simulink library "m3_common_lib"  (R2021b)
settings: Solver=ode45  StartTime=0.0  StopTime=10.0  RelTol=1e-3
undefined symbols (not defined in the file or in its folder): ACCEL_PRE_MULT, APDT_SrvcMgr_IRVHVDCSubFcnReq, C_C1GearNumbers, C_C1GearRatios, C_Calibration, C_DitherWaveform, C_GearOffset, C_GearRatioIn, C_GearRatioInverseOut, C_GearRatioOut, CLUTCH_INNER_LOOP_UPDATE_RATE, CONSTANT, DEGRADED_MODE_SIZE, Dem_EventStatusType, DiscIntNeverNeededParam, F_FAULT_ENUM, F_NOFAULT, F_OUTOFRANGE, F_RATELIMIT, FALSE, FMI14_SPECIAL_INSTRUCTIONS, FMI20_DATA_DRIFTED_HIGH, FMI21_DATA_DRIFTED_LOW, FMI29_RESERVED_FOR_SAE_ASSIGNMENT, FMI30_RESERVED_FOR_SAE_ASSIGNMENT, FMI31_CONDITION_EXISTS, FMI32_NO_FAULT, IC, k_accel, k_mean, MAX_UINT32, MEAN_PRE_MULT, NTriggers, QLTY_SIGNAL_FAILED, QLTY_SIGNAL_FULLY_FUNCTION, QLTY_SIGNAL_SUBSTITUTED_BY_1ST_CHOICE, QLTY_SIGNAL_SUBSTITUTED_BY_2ND_CHOICE, QLTY_SIGNAL_SUBSTITUTED_BY_3RD_CHOICE, QLTY_SIGNAL_SUBSTITUTED_BY_4TH_CHOICE, SAMPLE_TIME_100us, simin, T_TestPoint, TF_FALSE, TF_TRUE, TimeStep, TRUE, WORKSPACE_UPDATE_RATE, Zero, ZERO
libraries: $bdroot x121, simulink x23, simulink_extras x4, MBD_EPS_Local_Blockset x4
(part 2 of 10)

== system m3_common_lib/Diagnostics ==
  note: DEPRECATED
  note: Diagnostics
  note: DEPRECATED
  Calibration Enabled Debounce : Subsystem
      settings: RTWSystemCode=Inline
  Calibration Enabled Debounce Boolean Input : Subsystem
      settings: RTWSystemCode=Inline
  Calibration Enabled MinMax OOR : Subsystem  mask(Calibration Enabled OOR Detection Subsystem){InitialValue=0, InDataType=single}
      mask prompts: InitialValue "Initial Value"; InDataType "Input Data Type"
      mask init:
      | DataType = get_param(gcb, 'InDataType');
      | OOR = [gcb '/Enabled OOR'];
      | 
      | set_param(OOR, 'InDataType', DataType);
      mask TypeOptions InDataType: single | int16
  Calibration Enabled MinMax RLim : Subsystem  mask(Calibration Enabled RateLimit Detection Subsystem){IC=0, TimeStep=TimeStep, InDataType=single}
      mask prompts: IC "Initial Condition"; TimeStep "Update Time"; InDataType "Input Data Type"
      mask init:
      | DataType = get_param(gcb, 'InDataType');
      | RLim = [gcb '/Enabled RLim'];
      | 
      | set_param(RLim, 'InDataType', DataType);
      mask TypeOptions InDataType: single | int16
  Ccaller_DiagLv1 : Subsystem  TreatAsAtomicUnit=on
      settings: RTWSystemCode=Nonreusable function
  Ccaller_DiagLv2 : Subsystem  TreatAsAtomicUnit=on
      settings: RTWSystemCode=Nonreusable function
  DiagFaultCounter : Subsystem
  ExtractValue : Subsystem
      mask Display:
      | patch([0.3 0.3 0.7 0.7], [0.4 0.6 0.6 0.4], [205/255 205/255 255/255]);
      | disp('FromInputSignal')
      | port_label('input', 1, 'in');
      | port_label('output', 1, 'value');
      | port_label('output', 2, 'FMI');
  FMIUpdate : Subsystem
  Fault Debounce Lv1 Boolean Input : Subsystem
  Fault Debounce Lv1 state Input : Subsystem
  FaultStatusUpdate : Subsystem
  KeepAlive : Subsystem  TreatAsAtomicUnit=on  mask(KeepAlive){Operator===, UseSigObject=off}
      mask prompts: Operator "Relational Operator"; UseSigObject "Reuse Signal Object for Unit Delay"
      mask help:
      | Use to enable a subsystem that needs to keep itself alive based on a state created by the block.
      |
      | Enable = KeepAlive || (A (RelOp) B)
      |
      | Where RelOp can be any of the relational operators.
      | A and B must have the same data type.
      | All inputs must be scalars.
      |
      | Second output is the value of the (A (RelOp) B) which could be used in the enabled subsystem or for logging or terminated if unneeded.
      |
      | Checking "Reuse Signal Object for Unit Delay" is an optimization for when the signal driving KeepAlive is already a signal object.  Instead of allocating new memory for the unit delay, the unit delay will use the signal object.  In this case do not set the driving signal to "Resolve to Signal Object".
      mask init:
      | set_param([gcb '/RelOp'],'Operator',get_param(gcb,'Operator'));
      | 
      | ud = get_param([gcb '/Delay'],'Object');
      | if UseSigObject
      | st = get_param([gcb '/State'],'Object');
      | lh = st.PortHandles.Outport;
      | set(lh,'ShowPropagatedSignals','on');
      | set(lh,'ShowPropagatedSignals','off');
      | set(lh,'ShowPropagatedSignals','on');
      | sigName = get(lh,'PropagatedSignals');
      | ud.StateName = sigName;
      | ud.StateMustResolveToSignalObject = 'on';
      | else
      | ud.StateName = '';
      | ud.StateMustResolveToSignalObject = 'off';
      | end
      settings: RTWSystemCode=Inline
      mask TypeOptions Operator: == | ~= | < | <= | >= | >
      mask Display:
      | patch([0.3 0.3 0.7 0.7], [0.35 0.65 0.65 0.35], [255/255 127/255 255/255]);
      | 
      | if ~UseSigObject
      |    port_label('input',1,'KeepAlive');
      | else
      |    ph = get_param([gcb '/State'],'PortHandles');
      |    sigName = get(ph.Outport,'PropagatedSignals');
      |    port_label('input',1,['-E ' sigName]);
      | end
      | port_label('input',2,'A');
      | port_label('input',3,'B');
      | port_label('output',1,'Enable');
      | port_label('output',2,sprintf('(A %s B)',get_param(gcb,'Operator')));
  LogicBasedActivation : Subsystem  mask(AddDegradedMode){DM_SIZE=DEGRADED_MODE_SIZE}
      mask prompts: DM_SIZE "Degraded Mode Vector Size"
      mask help:
      | Logic based activation adds additional degraded modes if Add? input is true.  The logic can be disabled by the Enable input.
      |
      | - Enable: Allow or disallow logic.  Should be constant or calibration.
      | - DMToAdd: Packed degraded modes to add.  Size must match "Degraded Mode Vector Size" parameter.
      | - Add?: Boolean input to add DMs or pass through DMPackedData unchanged.
      | - DMPackedData: Current set of degraded modes.
      mask Display:
      | patch([0.3 0.3 0.7 0.7], [0.35 0.65 0.65 0.35], [255/255 127/255 255/255]);
      | port_label('input',1,'Enable');
      | port_label('input',2,'DMToAdd');
      | port_label('input',3,'Add?');
      | port_label('input',4,'DMPackedData');
      | port_label('output',1,'DMPackedData');
  LogicBasedDeactivation : Subsystem  mask(RemoveDegradedMode){DM_SIZE=DEGRADED_MODE_SIZE}
      mask prompts: DM_SIZE "Degraded Mode Vector Size"
      mask help:
      | Logic based deactivation removes degraded modes if Remove? input is true.  The logic can be disabled by the Enable input.
      |
      | - Enable: Allow or disallow logic.  Should be constant or calibration.
      | - DMToRemove: Packed degraded modes to remove.  Size must match "Degraded Mode Vector Size" parameter.
      | - Remove?: Boolean input to remove DMs or pass through DMPackedData unchanged.
      | - DMPackedData: Current set of degraded modes.
      mask Display:
      | patch([0.3 0.3 0.7 0.7], [0.35 0.65 0.65 0.35], [255/255 127/255 255/255]);
      | port_label('input',1,'Enable');
      | port_label('input',2,'DMToRemove');
      | port_label('input',3,'Remove?');
      | port_label('input',4,'DMPackedData');
      | port_label('output',1,'DMPackedData');
  OOR Fault Detect Enum : Subsystem  RTWFcnName=OOR  mask(CL OOR Fault Detection with Enable){InitialValue=0, k_min=0, k_max=0}
      mask prompts: InitialValue "Initial Value"; k_min "Lower Limit"; k_max "Upper Limit"
      mask help:
      | Out of range fault detection block with enable for Enum signals
      |
      | X(1) = input signal
      | X(2) = enable
      |
      | Y(1) = output signal
      | Y(2) = fault indication
      settings: RTWSystemCode=Inline  RTWFcnNameOpts=User specified  RTWFileNameOpts=Use function name
      mask Help: web(which(['common_lib12.html']))
      mask Display:
      | patch([0.1 0.1 0.9 0.9], [0.35 0.65 0.65 0.35], [255/255 127/255 255/255])
      | %disp('OOR/En')
      | 
      | min=get_param(gcb,'k_min')
      | max=get_param(gcb,'k_max')
      | 
      | txt = sprintf('\tUpper Lim: %s\n\tLower Lim: %s',max,min);
      | disp(txt)
      | 
      | port_label('input',1,'in')
      | port_label('input',2,'enable')
      | port_label('output',1,'out')
      | port_label('output',2,'fault?')
  OOR Fault Detection : Subsystem  RTWFcnName=OOR  mask(CL OOR Fault Detection with Enable){InitialValue=0, k_min=0, k_max=0, applyLimits=0}
      mask prompts: InitialValue "Initial Value"; k_min "Upper Limit"; k_max "Lower Limit"
      mask help:
      | Out of range fault detection block with enable
      |
      | X(1) = input signal
      | X(2) = enable
      |
      | Y(1) = saturated out
      | Y(2) = fault indication
      mask init:
      | portNumber = 1;
      | outMin = [];
      | outMax = [];
      | portHandles = get_param(gcb,'PortHandles');
      | inportHandle = portHandles.Inport(portNumber);
      | lineHandle = get_param(inportHandle,'Line');
      | if(lineHandle>0) 
      |     nvSrcPorts = get_param(lineHandle, 'NonVirtualSrcPorts');
      |     nvLineHandle = get_param(nvSrcPorts, 'line');
      |     if(nvLineHandle>0)
      |         nvSrcBlkHandle = get_param(nvLineHandle, 'SrcBlockHandle'); 
      |         blockTypeStr = get_param(nvSrcBlkHandle, 'BlockType');
      |         if(strcmp(blockTypeStr,'Inport')>0)
      |             outMin = get_param(nvSrcBlkHandle, 'OutMin');
      |             outMax = get_param(nvSrcBlkHandle, 'OutMax');
      |             set_param(gcb,'k_min',outMin);
      |             set_param(gcb,'k_max',outMax);
      |         else
      |             set_param(gcb,'k_min','0');
      |             set_param(gcb,'k_max','0');
      |             outMin = [];
      |             outMax = [];
      |         end
      |     else
      |         set_param(gcb,'k_min','0');
      |         set_param(gcb,'k_max','0');
      |         outMin = [];
      |         outMax = [];
      |     end
      | else
      |     set_param(gcb,'k_min','0');
      |     set_param(gcb,'k_max','0');
      |     outMin = [];
      |     outMax = [];
      | end
      | 
      | 
      | if isempty(outMin) || isempty(outMax) || ((strcmp(outMin,'0')>0)&&(strcmp(outMin,'0')>0))
      |     %applyLimits=false;
      |     set_param(gcb,'applyLimits','0')
      | else
      |     set_param(gcb,'applyLimits','1')
      | end
      settings: RTWSystemCode=Inline  RTWFcnNameOpts=User specified  RTWFileNameOpts=Use function name
      mask Help: web(which(['common_lib12.html']))
      mask DialogControl Control2 Prompt: Update
      mask DialogControl Control2 Callback:
      | portNumber = 1;
      | outMin = [];
      | outMax = [];
      | portHandles = get_param(gcb,'PortHandles');
      | inportHandle = portHandles.Inport(portNumber);
      | lineHandle = get_param(inportHandle,'Line');
      | if(lineHandle>0)
      |     nvSrcPorts = get_param(lineHandle, 'NonVirtualSrcPorts');
      |     nvLineHandle = get_param(nvSrcPorts, 'line');
      |     if(nvLineHandle>0)
      |         nvSrcBlkHandle = get_param(nvLineHandle, 'SrcBlockHandle');
      |         blockTypeStr = get_param(nvSrcBlkHandle, 'BlockType');
      |         if(strcmp(blockTypeStr,'Inport')>0)
      |             outMin = get_param(nvSrcBlkHandle, 'OutMin');
      |             outMax = get_param(nvSrcBlkHandle, 'OutMax');
      |             set_param(gcb,'k_min',outMin);
      |             set_param(gcb,'k_max',outMax);
      |         else
      |             set_param(gcb,'k_min','0');
      |             set_param(gcb,'k_max','0');
      |             outMin = [];
      |             outMax = [];
      |         end
      |     else
      |         set_param(gcb,'k_min','0');
      |         set_param(gcb,'k_max','0');
      |         outMin = [];
      |         outMax = [];
      |     end
      | else
      |     set_param(gcb,'k_min','0');
      |     set_param(gcb,'k_max','0');
      |     outMin = [];
      |     outMax = [];
      | end
      | 
      | if isempty(outMin) || isempty(outMax) || ((strcmp(outMin,'0')>0)&&(strcmp(outMin,'0')>0))
      |     %applyLimits=false;
      |     set_param(gcb,'applyLimits','0')
      | else
      |     set_param(gcb,'applyLimits','1')
      | end
      mask Display:
      | patch([0.1 0.1 0.9 0.9], [0.35 0.65 0.65 0.35], [255/255 127/255 255/255])
      | %disp('OOR/En')
      | 
      | min=get_param(gcb,'k_min')
      | max=get_param(gcb,'k_max')
      | 
      | txt = sprintf('\tUpper Lim: %s\n\tLower Lim: %s',max,min);
      | disp(txt)
      | 
      | port_label('input',1,'in')
      | port_label('input',2,'enable')
      | port_label('output',1,'out')
      | port_label('output',2,'fault?')
  SetFMI : Subsystem  mask(FMI_UPDATE){PRIORITY_1_FMI=FMI32_NO_FAULT, PRIORITY_2_FMI=FMI32_NO_FAULT, PRIORITY_3_FMI=FMI32_NO_FAULT, PRIORITY_4_FMI=FMI32_NO_FAULT, PRIORITY_5_FMI=FMI32_NO_FAULT, PRIORITY_6_FMI=FMI32_NO_FAULT, PRIORITY_7_FMI=FMI32_NO_FAULT}
      mask prompts: PRIORITY_1_FMI "Priority 1 FMI"; PRIORITY_2_FMI "Priority 2 FMI"; PRIORITY_3_FMI "Priority 3 FMI"; PRIORITY_4_FMI "Priority 4 FMI"; PRIORITY_5_FMI "Priority 5 FMI"; PRIORITY_6_FMI "Priority 6 FMI"; PRIORITY_7_FMI "Priority 7 FMI"
      mask help:
      | When no active FMI is present set the FMI according to the active inputs.
      |
      | If there are multiple active inputs, priority is assigned by input order.
      |
      | Unused inputs should be stubbed by ground blocks.  Corresponding FMI masked parameter should also be set to FMI32_NO_FAULT value for consistency.
      mask Display:
      | patch([0.3 0.3 0.7 0.7], [0.35 0.65 0.65 0.35], [255/255 127/255 255/255]);
      | port_label('input',1,'FMI');
      | port_label('input',2,sprintf('Set (%s)',get_param(gcb,'PRIORITY_1_FMI')));
      | port_label('input',3,sprintf('Set (%s)',get_param(gcb,'PRIORITY_2_FMI')));
      | port_label('input',4,sprintf('Set (%s)',get_param(gcb,'PRIORITY_3_FMI')));
      | port_label('input',5,sprintf('Set (%s)',get_param(gcb,'PRIORITY_4_FMI')));
      | port_label('input',6,sprintf('Set (%s)',get_param(gcb,'PRIORITY_5_FMI')));
      | port_label('input',7,sprintf('Set (%s)',get_param(gcb,'PRIORITY_6_FMI')));
      | port_label('input',8,sprintf('Set (%s)',get_param(gcb,'PRIORITY_7_FMI')));
      | port_label('output',1,'FMI');
  SignalSubstitution : Subsystem  TreatAsAtomicUnit=on  mask(SignalSubstitution){}
      mask help:
      | Output first non-faulted signal or in the case of all faulted, output the failed value input.
      |
      | Quality will have a value between 0 and 100 dropping from 100 in increments of 20 for each faulted signal.
      settings: RTWSystemCode=Inline
      mask Display:
      | patch([0.3 0.3 0.7 0.7], [0.35 0.65 0.65 0.35], [255/255 127/255 255/255]);
      | port_label('input',1,'Signal');
      | port_label('input',2,'Signal Faulted');
      | port_label('input',3,'1st Choice');
      | port_label('input',4,'1st Choice Faulted');
      | port_label('input',5,'2nd Choice');
      | port_label('input',6,'2nd Choice Faulted');
      | port_label('input',7,'3rd Choice');
      | port_label('input',8,'3rd Choice Faulted');
      | port_label('input',9,'4th Choice');
      | port_label('input',10,'4th Choice Faulted');
      | port_label('input',11,'Failed Value');
      | port_label('output',1,'Signal');
      | port_label('output',2,'Quality');
  SpeedRationalityFaultDetect : Subsystem
  ToRWSignal : Subsystem
      mask Display:
      | patch([0.3 0.3 0.7 0.7], [0.4 0.6 0.6 0.4], [205/255 205/255 255/255]);
      | disp('ToInputSignal')
      | port_label('input', 1, 'in');
      | port_label('input', 2, 'FMI');
      | port_label('output', 1, 'out');

== system m3_common_lib/Documentation ==
  note: Documentation
  EatonLogo : Subsystem
      mask Display: image('EatonLogo.jpg')
  LegalNoticeEaton : Subsystem  mask(LegalNotice){Company=Eaton Corporation}
      mask prompts: Company "Select Company"
      mask TypeOptions Company: Eaton Corporation | Eaton Cummins Automated Transmission Technologies
      mask Display:
      | corp = get_param(gcb,'Company');
      | disp(sprintf([...
      | 'Unpublished Work\n',...
      | 'Copyright %s %s.\n',...
      | 'Notice:\n',...
      | 'This document contains confidential information.\n',...
      | 'Disclosure of this information is conditioned upon the recipient''s agreement that\n',...
      | 'the use of the information shall be only for the purpose motivating the disclosure.\n',...
      | 'Any other use is strictly prohibited without the prior written consent.'],...
      | datestr(now,'yyyy'),corp))
  RequirementLinks : Subsystem  mask(ReqLink){}
      settings: OpenFcn=open_system([gcb '/DocBlock'])
      mask Display:
      | a = get_param([gcb '/DocBlock'],'UserData');
      | if isempty(a)
      |     disp('Double Click to Open');
      | else
      |     disp(sprintf('Requirements (REQ_####)\n%s',a.content));
      | end
  SubsystemPath : Subsystem  mask(SubSysPathInfo){}
      mask Display: disp(regexprep(get_param(gcb,'parent'),'/','>'))

== system m3_common_lib/Fltrs ==
  note: Filters
  Fltr : Subsystem  RTWFcnName=FLTR  mask(CL Filter){TimeStep=[]}
      mask prompts: TimeStep "Time Step"
      mask help:
      | First Order Filter, y(n)= T/tau x(n) + (1 - T/tau) y(n-1)
      |
      | output = previous output + (input - previous output) * T/tau
      |
      | X(1) = input
      | X(2) = tau
      |
      | Y(1) = output
      |
      | Time step is entered via mask parameter.
      | NgEK, Inc.
      mask init:
      | %switch class(TimeStep)
      | %   case ('double')
      | %      IC = double(0.0);
      | %   case ('single')
      |        IC = single(0.0);
      | %   case ('int8')
      | %      IC = int8(0);
      | %   case ('int16')
      | %      IC = int16(0);
      | %   case ('int32')
      | %      IC = int32(0);
      | %end;
      | Ts = single(TimeStep);
      settings: RTWFcnNameOpts=User specified  RTWFileNameOpts=Use function name
      mask Help: web(which(['common_lib16.html']))
      mask Display:
      | patch([0.35 0.35 0.65 0.65], [0.4 0.6 0.6 0.4], [255/255 127/255 255/255])
      | disp('Filter')
      | port_label('input', 1, 'input')
      | port_label('input', 2, 'tau')
      | port_label('output', 1, 'output')
  Fltr_wR : Subsystem  mask(CL Filter wRO){TimeStep=[]}
      mask prompts: TimeStep "Time Step"
      mask help:
      | First Order Filter, y(n)= T/tau x(n) + (1 - T/tau) y(n-1)
      |
      | If      reset is true (1) then output=initial condition
      |    otherwise output = previous output + (input - previous output) * T/tau
      |
      | X(1) = input
      | X(2) = tau
      | X(3) = initial condition
      | X(4) = reset flag
      |
      | Y(1) = output
      |
      | Time step is entered via mask parameter.
      | NgEK, Inc.
      mask init: same as m3_common_lib/Fltrs/Fltr
      mask Help: web(which(['common_lib18.html']))
      mask Display:
      | patch([0.4 0.4 0.6 0.6], [0.35 0.65 0.65 0.35], [255/255 127/255 255/255])
      | disp('Filter\nw R')
      | port_label('input', 1, 'input')
      | port_label('input', 2, 'tau')
      | port_label('input', 3, 'ic')
      | port_label('input', 4, 'reset?')
      | port_label('output', 1, 'output')
  Fltr_wRO : Subsystem  RTWFcnName=FLTRWRO  mask(CL Filter wRO){TimeStep=[]}
      mask prompts: TimeStep "Time Step"
      mask help:
      | First Order Filter, y(n)= T/tau x(n) + (1 - T/tau) y(n-1)
      |
      | If override is true (1) then output=override_value
      | If      reset is true (1) then output=input
      |    otherwise output = previous output + (input - previous output) * T/tau
      |
      | X(1) = input
      | X(2) = tau
      | X(3) = override value
      | X(4) = override flag
      | X(5) = reset flag
      |
      | Y(1) = output
      |
      | Time step is entered via mask parameter.
      | NgEK, Inc.
      mask init:
      | %switch class(TimeStep)
      | % case ('double')
      | %      IC = double(0.0);
      | %    case ('single')
      |        IC = single(0.0);
      | %    case ('int8')
      | %         IC = int8(0);
      | %    case ('int16')
      | %      IC = int16(0);
      | %   case ('int32')
      | %        IC = int32(0);
      | %end;
      | Ts = single(TimeStep);
      settings: RTWFcnNameOpts=User specified  RTWFileNameOpts=Use function name
      mask Help: web(which(['common_lib17.html']))
      mask Display:
      | patch([0.4 0.4 0.6 0.6], [0.35 0.65 0.65 0.35], [255/255 127/255 255/255])
      | disp('Filter\nw RO')
      | port_label('input', 1, 'input')
      | port_label('input', 2, 'tau')
      | port_label('input', 3, 'override_value')
      | port_label('input', 4, 'override?')
      | port_label('input', 5, 'reset?')
      | port_label('output', 1, 'output')
  Fltr_wROExtInitCond : Subsystem  TreatAsAtomicUnit=on  RTWFcnName=FLTRWRO  mask(CL Filter wRO wIC){TimeStep=[]}
      mask prompts: TimeStep "Time Step"
      mask help:
      | First Order Filter, y(n)= T/tau x(n) + (1 - T/tau) y(n-1)
      |
      | If override is true (1) then output=override_value
      | If      reset is true (1) then output=input
      |    otherwise output = previous output + (input - previous output) * T/tau
      |
      | X(1) = input
      | X(2) = tau
      | X(3) = inititial condition
      | X(4) = reset
      | X(5) = override TO
      | X(6) = override value TC
      | Y(1) = output
      mask init:
      | %switch class(TimeStep)
      | % case ('double')
      | %      IC = double(0.0);
      | %    case ('single')
      | %       IC = single(0.0);
      | %    case ('int8')
      | %         IC = int8(0);
      | %    case ('int16')
      | %      IC = int16(0);
      | %   case ('int32')
      | %        IC = int32(0);
      | %end;
      | %task_rate = single(taskrate_input);
      | Ts = single(TimeStep);
      settings: RTWFcnNameOpts=User specified  RTWFileNameOpts=Use function name
      mask Help: web(which(['common_lib17.html']))
      mask Display:
      | patch([0.2 0.2 0.8 0.8], [0.35 0.65 0.65 0.35], [255/255 127/255 255/255])
      | disp('Filter\n w ROExtInitCond')
      | port_label('input', 1, 'input')
      | port_label('input', 2, 'tau')
      | port_label('input', 3, 'ic')
      | port_label('input', 4, 'reset?')
      | port_label('input', 5, 'override?')
      | port_label('input', 6, 'override_value')
      | port_label('output',1, 'output')
  Int16FIR : Subsystem  mask(FIRInt16){N=50, Ts=0.01}
      mask prompts: N "Half Window Size (samples)"; Ts "Time Step"
      mask help:
      | Highly optimized FIR filter designed to calculated mean and least squares fit slope.
      |
      | For best results scale the input to use the whole range of int16, but note acceleration can saturate.  The buffer initializes to zero.
      |
      | Termination of an output will eliminate relevant code to calculate that output.
      mask init:
      | [k_mean, MEAN_PRE_MULT, k_accel, ACCEL_PRE_MULT] = FixedPointFIRInit(N,Ts);
      mask Display:
      | patch([0.35 0.35 0.65 0.65], [0.4 0.6 0.6 0.4], [255/255 127/255 255/255])
      | disp('Int16 FIR')
      | port_label('input', 1, 'u')
      | port_label('output', 1, 'mean')
      | port_label('output', 2, 'accel')
  Inv_Fltr : Subsystem  mask(CL Inverse Filter){TimeStep=[]}
      mask prompts: TimeStep "Time Step"
      mask help:
      | Inverse First Order Filter
      | u(k) = y(k-1) + tau/TimeStep*(y(k) - y(k-1))
      |
      | X(1) = input
      | X(2) = tau
      |
      | Y(1) = output
      |
      | Time step is entered via mask parameter.
      | NgEK, Inc.
      mask init:
      | %switch class(TimeStep)
      | %   case ('double')
      | %      Zero = double(0.0);
      | %   case ('single')
      |        Zero = single(0.0);
      | %   case ('int8')
      | %      Zero = int8(0);
      | %   case ('int16')
      | %      Zero = int16(0);
      | %   case ('int32')
      | %      Zero = int32(0);
      | %end;
      mask Help: web(which(['common_lib47.html']))
      mask Display:
      | patch([0.35 0.35 0.65 0.65], [0.3 0.7 0.7 0.3], [255/255 127/255 255/255])
      | disp('Inverse\nFilter')
      | port_label('input', 1, 'input')
      | port_label('input', 2, 'tau')
      | port_label('output', 1, 'output')
  Inv_RpdFltr : Subsystem  mask(CL Inverse Rapid Filtering){DType=Single}
      mask prompts: DType "Data Type"
      mask help:
      | Inverse of the Rapid Filter.  u(k) = y(k-1) + (y(k) - y(k-1))/fc
      |
      | X(1) = input
      | X(2) = filter constant
      |
      | Y(1) = output
      | NgEK, Inc.
      mask init:
      | switch class(TimeStep)
      |     case ('double')
      |         Zero = double(0.0);
      |     case ('single')
      |         Zero = single(0.0);
      |     case ('int8')
      |         Zero = int8(0);
      |     case ('int16')
      |         Zero = int16(0);
      |     case ('int32')
      |         Zero = int32(0);
      | end;
      mask Help: web(which(['common_lib48.html']))
      mask TypeOptions DType: Double | Single | Int8 | Int16 | Int32
      mask Display:
      | patch([0.30 0.30 0.70 0.70], [0.25 0.75 0.75 0.25], [255/255 127/255 255/255])
      | disp('Inverse\nRapid\nFiltering')
      | port_label('input', 1, 'input')
      | port_label('input', 2, 'fltr_cnst')
      | port_label('output', 1, 'output')
  Lookup_wFltr : Subsystem  mask(CL Filter wRO wIC wLut){TimeStep=[], Mode=Linear Interpolation}
      mask prompts: TimeStep "Time Step"; Mode "Interpolation Mode"
      mask help:
      | This block combines a 2D Table lookup with explicit axis inputs with a First Order Filter.
      |
      | First Order Filter, y(n)= T/tau x(n) + (1 - T/tau) y(n-1)
      |
      | If override is true (1) then output=override_value
      | If reset is true (1) then output=lookup_table_interpolation
      |    otherwise output = previous output + (lookup_table_interpolation - previous output) * T/tau
      |
      | X(1) = Independent variable
      | X(2) = X axis vector
      | X(3) = Y axis vector
      | X(4) = Override TO
      | X(5) = Override value TC
      | X(6) = Filter enable
      | X(7) = Filter tau
      | X(8) = Filter initial condition
      | Y(1) = Output
      |
      | Interpolation mode is selected via the mask:
      |
      | Ceiling Interpolation: rounds up in the positive direction
      | Floor Interpolation: rounds down in the negative direction
      | Nearest (Neighbor) Interpolation: rounds to the closest representable number
      | Linear Interpolation: Interpolates data by assuming data varies linearly between points
      mask init: same as m3_common_lib/Fltrs/Fltr_wROExtInitCond
      mask TypeOptions Mode: Linear Interpolation | Nearest Neighbor | Floor | Ceiling
      mask Display:
      | patch([0.30 0.30 0.70 0.70], [0.45 0.55 0.55 0.45], [255/255 127/255 255/255])
      | disp('Lookup_wFltr')
      | port_label('input', 1, 'input')
      | port_label('input', 2, 'x-axis vector')
      | port_label('input', 3, 'y-axis vector' )
      | port_label('input', 4, 'override?')
      | port_label('input', 5, 'override_value')
      | port_label('input', 6, 'filter_enable?')
      | port_label('input', 7, 'tau')
      | port_label('input', 8, 'ic')
      | port_label('output', 1, 'output')
  Rpd_Fltr : Subsystem  mask(CL Rapid Filter){DType=Single}
      mask prompts: DType "Data Type"
      mask help:
      | Rapid 1st Order Filter, y(k)=x(k) + Fc*( Y(k-1) - X(k) )
      |
      | X(1) = input
      | X(2) = filter constant
      |
      | Y(1) = output
      | NgEK, Inc.
      mask init:
      | switch DType
      |    case (1)
      |        IC = double(0.0);
      |   case (2)
      |        IC = single(0.0);
      |    case (3)
      |          IC = int8(0);
      |     case (4)
      |          IC = int16(0);
      |    case (5)
      |        IC = int32(0);
      | end;
      mask Help: web(which(['common_lib19.html']))
      mask TypeOptions DType: Double | Single | Int8 | Int16 | Int32
      mask Display:
      | patch([0.35 0.35 0.65 0.65], [0.35 0.65 0.65 0.35], [255/255 127/255 255/255])
      | disp('Rapid\nFilter')
      | port_label('input', 1, 'input')
      | port_label('input', 2, 'fltr_cnst')
      | port_label('output', 1, 'output')
  Scaling_wFltr : Subsystem  mask(CL Filter wRO wIC wScl){TimeStep=[]}
      mask prompts: TimeStep "Time Step"
      mask help:
      | This block adds sclaing to scale the raw input signal. The signal is then filtered using first order filter.
      |
      | First Order Filter, y(n)= T/tau x(n) + (1 - T/tau) y(n-1)
      |
      | If override is true (1) then output=override_value
      | If reset is true (1) then output=input*resolution+offset
      |    otherwise output = previous output + ((input*resolution+offset) - previous output) * T/tau
      |
      | X(1) = input
      | X(2) = resolution
      | X(3) = offset
      | X(4) = override TO
      | X(5) = override value TC
      | X(6) = filter enable
      | X(7) = filter tau
      | X(8) = filter initial condition
      | Y(1) = output
      mask init: same as m3_common_lib/Fltrs/Fltr_wROExtInitCond
      mask Display:
      | patch([0.30 0.30 0.70 0.70], [0.45 0.55 0.55 0.45], [255/255 127/255 255/255])
      | disp('Scaling_wFltr')
      | port_label('input', 1, 'input')
      | port_label('input', 2, 'res')
      | port_label('input', 3, 'offset' )
      | port_label('input', 4, 'override?')
      | port_label('input', 5, 'override_value')
      | port_label('input', 6, 'filter_enable?')
      | port_label('input', 7, 'tau')
      | port_label('input', 8, 'ic')
      | port_label('output', 1, 'output')

== system m3_common_lib/Fuzzy ==
  note: Fuzzy Controller Design
  Demux : Demux  Outputs=2
  Fuzzy Implication : Subsystem  mask(CL Fuzzy Implication){from=ShiftPoint, value=HighUpshiftPoint}
      mask prompts: from "Result Bus Goto Tag"
      mask help:
      | The fuzzy implication is the final result of a decision tree branch.
      |
      | The value parameter of this block selects from the Result Bus the particular value that the output should take on when the associated branch is true.
      |
      | It is ok and likely to have multiple branches that result in the same value.  Adding all the result branches together will give a weight sum of the result.
      mask init:
      | set_param([gcb '/From'],'GotoTag',get_param(gcb,'from'));
      | set_param([gcb '/Select'],'OutputSignals',get_param(gcb,'value'))
      mask Display:
      | patch([0.25 0.25 0.75 0.75], [0.25 0.75 0.75 0.25], [255/255 127/255 255/255])
      | port_label('input',1,'THEN');
      | disp([get_param(gcb,'from') ' is\n' get_param(gcb,'value')])
  Fuzzy Intersection : Subsystem  mask(CL Fuzzy Decision){from=DataBus, signal=Demand, value=value, dispStr=Demand is\nvalue}
      mask prompts: from "Data Bus Goto Tag"; signal "Signal Name"; value "Value(s) (Comma seperated list of named values)"
      mask help:
      | The Fuzzy Decision block serves as the fuzzy AND operator.
      |
      | Input - Truth of previous statements.
      | TRUE Output - Incoming truth AND truth of selected signal values(s).
      | FALSE Output - Incoming truth AND falseness of selected signal values(s).
      |
      | TRUE Output + FALSE Output = Input
      mask init:
      | fromDlg = get_param(gcb,'from');
      | fromBlk = get_param([gcb '/From'],'GotoTag');
      | if ~strcmp(fromDlg,fromBlk)
      |    set_param([gcb '/From'],'GotoTag',get_param(gcb,'from'));
      | end
      | 
      | remain = strtrim(get_param(gcb,'value'));
      | first = true;
      | output = '';
      | sig = get_param(gcb,'signal');
      | dstr = [sig ' is\n'];
      | while any(remain)
      |     [str, remain] = strtok(remain,{',',' '});
      |     if first
      |         output = [sig '.' str];
      |         dstr = [dstr str];
      |     else
      |         output = [output ',' sig '.' str];
      |         dstr = [dstr '\nOR ' str];
      |     end
      |     first = false;
      | end
      | 
      | if ~strcmp(get_param(gcb,'dispStr'),dstr) || ...
      |    ~strcmp(get_param([gcb '/Select'],'OutputSignals'),output)
      |    set_param(gcb,'dispStr',dstr);
      | 
      |    %Delete old lines
      |    sel = get_param([gcb '/Select'],'PortHandles');
      |    n = length(sel.Outport);
      |    for i = 1:n
      |        line = get(sel.Outport(i),'Line');
      |        if line>0
      |            delete_line(line);
      |        end
      |    end
      | 
      |    %Set the new outputs
      |    set_param([gcb '/Select'],'OutputSignals',output)
      | 
      |    %Add new lines
      |    sel = get_param([gcb '/Select'],'PortHandles');
      |    n = length(sel.Outport);
      |    set_param([gcb '/OR'],'Inputs',char(ones(1,n)*'+'));
      |    for i = 1:n
      |        istr = num2str(i);
      |        add_line(gcb,['Select/' istr],['OR/' istr]);
      |    end
      | end
      mask Help:
      | The Fuzzy Decision block serves as the fuzzy AND operator.  The TRUE output
      | is the truth of the input AND truth of the selected signal value(s).  The
      | FALSE output is truth of the input but falseness of the selected signal
      | value(s).  Thus the sum of TRUE and FALSE output will equal the truth of
      | the input.
      | 
      | Use this block as nodes in a binary decision tree.  The root node should
      | always have an input truth of 1.0, the sum of all branches.  At the end of
      | each branch should be a Fuzzy THEN statement followed by a summation of all
      | THEN statements.
      mask Callback value:
      | if isempty(strtrim(get_param(gcb,'value')))
      |     set_param(gcb,'value','value');
      | end
      mask Display:
      | patch([0.25 0.25 0.75 0.75], [0.25 0.75 0.75 0.25], [255/255 127/255 255/255])
      | port_label('input',1,'IF');
      | port_label('output',1,'THEN');
      | port_label('output',2,'ELSE');
      | disp(get_param(gcb,'dispStr'))
  Fuzzy Membership Function : Subsystem  mask(CL Fuzzy Membership){}
      mask help:
      | This fuzzy membership function uses triangular functions centered at the breakpoints defined by the second input.  A ramp function is used for the first and last break point.
      |
      | This membership function enforces the property of mutual exclusivity.  The sum of all memberships equals 1.0 for the range of the input.
      |
      | The breakpoints must be in increasing order and be unique.  If not, order and uniqueness will be enforced by shifting breakpoints above the previously listed value in an iterative fasion.
      |
      | First Input - Input signal
      | Second Input - Breakpoint list
      mask Display:
      | patch([0.22 0.22 0.8 0.8], [0.3 0.68 0.68 0.3], [255/255 127/255 255/255])
      | plot([0.0 0.4 0.4],[0.8 0.8 0.7]);
      | text(0.15,0.65,'1');
      | plot([0.2 0.3 0.5 0.8],[0.7 0.7 0.3 0.3]);
      | plot([0.3 0.5 0.7],[0.3 0.7 0.3]);
      | text(0.15,0.35,'0');
      | plot([0.2 0.5 0.7 0.8],[0.3 0.3 0.7 0.7]);
      | 
      | 
      | plot([0.0 0.3 0.3 0.3 0.5 0.5 0.5 0.7 0.7],[0.2 0.2 0.25 0.2 0.2 0.25 0.2 0.2 0.25])
  Fuzzy Union : Sum  Inputs=|++
  Goto Tag Visibility : GotoTagVisibility  GotoTag=DataBus
  Goto Tag Visibility1 : GotoTagVisibility  GotoTag=ResultBus
  Truth : Constant  Value=single(1.0)  SampleTime=-1

== system m3_common_lib/Gear Ratios ==
  note: Gear Ratios
  FindGearNumberByRatio : Subsystem  mask{RatioToGearIn=C_C1GearRatios, RatioToGearOut=C_C1GearNumbers, GearToRatioIn=C_GearRatioIn, GearToRatioOut=C_GearRatioOut, ConfirmTime=single(0), TimeStep=0.001}
      mask prompts: RatioToGearIn "RatioToGearIn (single)"; RatioToGearOut "RatioToGearOut (single)"; GearToRatioIn "GearToRatioIn (single)"; GearToRatioOut "GearToRatioOut (single)"; ConfirmTime "Speeed Confirmation Time (single)"; TimeStep "Time Step (double)"
      mask help:
      | This block outputs the GearNumber closest to the ratio appearing at the
      | input.  The block requires monotonically increasing tables.  i.e. the
      | RatioToGearIn and GearToRatioIn values must be increasing.
      |
      | The block works for both forward and reverse ratios.  (Positive and negative
      | speed and ratio).
      |
      | GearNumber - The gear number of the determined ratio.  Set to single(0) if
      | ratio does not match an available ratio.
      |
      | OutputValid - True if the ratio matches for ConfirmTime and above MinSpeed.
      |
      | SpeedAboveMin - True if speed is above MinSpeed.
      |
      | Ratio = ClutchSpeed/OutputSpeed
  GearNumberToRatio : Subsystem
      mask Display:
      | patch([0.3 0.3 0.7 0.7], [0.4 0.6 0.6 0.4], [255/255 127/255 255/255]);
      | disp('Gear Num\n to Ratio')
      | port_label('input',1,'gear_num')
      | port_label('output',1,'ratio')
      | port_label('output',2,'inv_ratio')

== system m3_common_lib/IO ==
  note: IO Blocks
  Calibration with Pretty Print Value : Subsystem  mask(Calibratible Input){CalValue=C_Calibration, scaling=None}
      mask prompts: CalValue "Calibratible Name"
      mask help:
      | This block is simply a standard Simulink constant block w/ a custom wrapper to pretty-print the calibratible value on the mask.
      |
      | NgEK, Inc.
      mask init:
      | CalName = get_param(gcb,'CalValue');
      mask TypeOptions scaling: None | RPM | MPH
      mask Display:
      | fprintf([CalName ' = ' num2str(double(CalValue)*...
      |     (strcmp(get_param(gcb,'scaling'),'RPM')*30/pi+...
      |      strcmp(get_param(gcb,'scaling'),'MPH')*2.236936292+...
      |      strcmp(get_param(gcb,'scaling'),'None')*1.0)) ' '...
      |      char(strcmp(get_param(gcb,'scaling'),'RPM')*double('RPM')+...
      |           strcmp(get_param(gcb,'scaling'),'MPH')*double('MPH')+...
      |           strcmp(get_param(gcb,'scaling'),'None')*double(sprintf('   ')))])
  Calibration with Pretty Print Value1 : $bdroot/IO/Calibration with Pretty Print Value  CalValue=c_Calibration  scaling=None
  From Workspace w/Datatype : Subsystem  mask(From Workspace w/Datatype){st=0, var=simin, intdat=on, zerocross=off, extmode=Extrapolation}
      mask prompts: st "sample time"; var "data"; intdat "Interpolate data"; zerocross "Enable zero crossing detection"; extmode "Form output after final data value by:"
      mask help:
      | From worspace block with data type convertor at its output.
      |
      | NgEK, Inc.
      mask init:
      | dt = get_param(gcb,'st');
      | data = get_param(gcb,'var');
      | blk = [gcb '/From' sprintf('\n') 'Workspace'];
      | if intdat, mode = 'on'; else mode = 'off'; end
      | set_param(blk,'interpolate',mode)
      | if zerocross, mode = 'on'; else mode = 'off'; end
      | set_param(blk,'zerocross',mode)
      | switch extmode
      |     case 1
      |         mode = 'Extrapolation';
      |     case 2
      |         mode = 'Setting to zero';
      |     case 3
      |         mode = 'Hold final value';
      |     case 4
      |         mode = 'Cyclic repetition';
      | end
      | set_param(blk,'outputafterfinalvalue',mode)
      mask Help: Use just like the original from workspace block.
      mask TypeOptions extmode: Extrapolation | Setting to zero | Holding final value | Cyclic repetition
      mask Display: disp(data)
  Triangle : Subsystem  mask(CL Triangle){TimeStep=[]}
      mask prompts: TimeStep "Time Step"
      mask help:
      | Output a triangle signal of specified amplitude, offset and frequency.
      |
      | X(1) = amplitude
      | X(2) = frequency
      | X(3) = offset
      |
      | Y(1) = output
      |
      | Time step is entered via mask parameter.
      | NgEK, Inc.
      mask init:
      | h=[gcb '/Data Type Conversion'];
      | 
      | %switch class(TimeStep)
      | %   case ('double')
      | %      Zero        = double( 0.0);
      | %      ZeroZeroOne = double( 0.001);
      | %      One         = double( 1.0);
      | %      Two         = double( 2.0);
      | %      MinusOne    = double(-1.0);
      | %      set_param(h, 'DataType','double');
      | %      set_param([h '1'], 'DataType','double');
      | %   case ('single')
      |        Zero        = single( 0.0);
      |        ZeroZeroOne = single( 0.001);
      |        One         = single( 1.0);
      |        Two         = single( 2.0);
      |        MinusOne    = single(-1.0);
      |        set_param(h, 'DataType','single');
      |        set_param([h '1'], 'DataType','single');
      | %end;
      mask Help: web(which(['common_lib20.html']))
      mask Display:
      | patch([0.375 0.375 0.625 0.625], [0.35 0.65 0.65 0.35], [255/255 127/255 255/255])
      | plot([0.375 0.4375 .5 0.5625 0.625],[0.35 0.65 0.35 0.65 0.35]);
      | port_label('input', 1, 'amplitude')
      | port_label('input', 2, 'frequency')
      | port_label('input', 3, 'offset')
      | port_label('output', 1, 'output')

== system m3_common_lib/Integrators ==
  note: Integrators
  ForwardEulerIntergrator : Subsystem  mask{IC=0, TSAMP=0}
      mask prompts: IC "Initial Condition"; TSAMP "Sample Time"
      mask Display:
      | patch([0.35 0.35 0.65 0.65], [0.3 0.7 0.7 0.3], [255/255 127/255 255/255])
      | disp('Forward Euler\nIntegral')
      | port_label('input',1,'dx')
      | port_label('input',2,'x0')
      | port_label('input',3,'reset')
      | port_label('output',1,'x')
